simulink library "magField_custom_lib"  (R2018b)
settings: Solver=VariableStepAuto  StartTime=0.0  StopTime=10.0  RelTol=1e-3
settings Model: Creator=Taylor  LastModifiedBy=Taylor

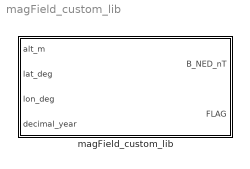
== system magField_custom_lib ==
  magField_custom_lib : Subsystem

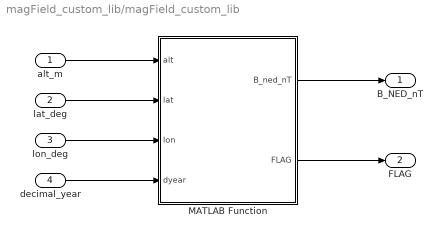
== system magField_custom_lib/magField_custom_lib ==
  alt_m : Inport
  lat_deg : Inport  Port=2
  lon_deg : Inport  Port=3
  decimal_year : Inport  Port=4
  MATLAB Function : MATLAB Function  TreatAsAtomicUnit=on
  B_NED_nT : Outport
  FLAG : Outport  Port=2
  wires:
  decimal_year/1 -> MATLAB Function/4(dyear)
  lon_deg/1 -> MATLAB Function/3(lon)
  lat_deg/1 -> MATLAB Function/2(lat)
  alt_m/1 -> MATLAB Function/1(alt)
  MATLAB Function/1(B_ned_nT) -> B_NED_nT/1
  MATLAB Function/2(FLAG) -> FLAG/1

== matlab function magField_custom_lib/MATLAB Function ==
  data: alt input; lat input; B_ned_nT output; lon input; dyear input; FLAG output
function [B_ned_nT,FLAG]  = my_wmm(alt,lat,lon,dyear)
%MY_WMM   World Magnetic Model
%
% B_NED_nT = my_wmm(lat,lon,alt,dyear) returns the magnetic field vector at
% the current latitude, longitude and altitude at the time specified by the 
% input dyear (decimal year). LLA can (should) be the output of the matlab
% function ecef2lla.m to make things simple. 
%
% Inputs:
%   - lat : geodetic latitude [degrees]
%   - lon : geodetic longitude [degrees]
%   - alt : altitude above the WGS84 ellipsoid [km]
%   - dyear : decimal year (e.g. 2016.25) MUST be greater than 2015.0
%
% Outputs: 
%   - B_ned_nT : magnetic field vector in the North-East-Down frame with
%   units of nanoTesla.
%   - FLAG : exit flag that indicates an error (-1) if the year is out of
%   range, otherwise this is 0.
%
% Current coefficients: WMM 2015v2 -- see Include/WMM_2015v2.COF file
% NOAA publishes user manuals, coefficient files and some software on their
% webiste here: https://www.ngdc.noaa.gov/geomag/WMM/soft.shtml#downloads
% This function was built from the WMM2015_Report.pdf 
%
% T. Reynolds -- RAIN Lab

%#codegen

% Constants
A       = 6378137;          % semi major axis [m]
a       = 6371200;          % geomagnetic reference radius
f       = 1/298.257223563;  % reciprocal flatening
e2      = f*(2-f);          % eccentricity squared
ord     = 12;               % model order 
maxord  = ord+1;
DEG2RAD = pi/180;

% HARD CODED COEFFICIENTS
t0 = 2015.0;
g = [ -29438.2, -1493.5,      0,      0,      0,     0,     0,     0,    0,     0,    0,    0, 0;
       -2444.5,  3014.7,   1679,      0,      0,     0,     0,     0,    0,     0,    0,    0, 0;
        1351.8, -2351.6, 1223.6,  582.3,      0,     0,     0,     0,    0,     0,    0,    0, 0;
         907.5,   814.8,  117.8, -335.6,   69.7,     0,     0,     0,    0,     0,    0,    0, 0;
        -232.9,   360.1,  191.7, -141.3, -157.2,   7.7,     0,     0,    0,     0,    0,    0, 0;
          69.4,    67.7,   72.3, -129.1,  -28.4,  13.6, -70.3,     0,    0,     0,    0,    0, 0;
          81.7,   -75.9,   -7.1,   52.2,   15,     9.1,    -3,   5.9,    0,     0,    0,    0, 0;
          24.2,     8.9,  -16.9,   -3.1,  -20.7,  13.3,  11.6, -16.3, -2.1,     0,    0,    0, 0;
           5.5,     8.8,      3,   -3.2,    0.6, -13.2,  -0.1,   8.7, -9.1, -10.4,    0,    0, 0;
            -2,    -6.1,    0.2,    0.6,   -0.5,   1.8,  -0.7,   2.2,  2.4,  -1.8, -3.6,    0, 0;
             3,    -1.4,   -2.3,    2.1,   -0.8,   0.6,  -0.7,   0.1,  1.7,  -0.2,  0.4,  3.5, 0;
            -2,    -0.1,    0.5,    1.2,   -0.9,   0.9,   0.1,   0.6, -0.4,  -0.5,  0.2, -0.9, 0 ];
     
h = [ 0,  4796.3,      0,      0,     0,     0,     0,    0,    0,    0,    0,    0, 0;
      0, -2842.4, -638.8,      0,     0,     0,     0,    0,    0,    0,    0,    0, 0;
      0,  -113.7,  246.5, -537.4,     0,     0,     0,    0,    0,    0,    0,    0, 0;
      0,   283.3, -188.6,  180.7,  -330,     0,     0,    0,    0,    0,    0,    0, 0;
      0,    46.9,  196.5, -119.9,    16, 100.6,     0,    0,    0,    0,    0,    0, 0;
      0,   -20.1,   32.8,   59.1, -67.1,   8.1,  61.9,    0,    0,    0,    0,    0, 0;
      0,   -54.3,  -19.5,      6,  24.5,   3.5, -27.7, -2.9,    0,    0,    0,    0, 0;
      0,    10.1,  -18.3,   13.3, -14.5,  16.2,     6, -9.2,  2.4,    0,    0,    0, 0;
      0,   -21.8,   10.7,   11.8,  -6.8,  -6.9,   7.9,    1, -3.9,  8.5,    0,    0, 0;
      0,     3.3,   -0.4,    4.6,   4.4,  -7.9,  -0.6, -4.2, -2.9, -1.1, -8.8,    0, 0;
      0,       0,    2.1,   -0.6,  -1.1,   0.7,  -0.2, -2.1, -1.5, -2.6,   -2, -2.3, 0;
      0,      -1,    0.3,    1.8,  -2.2,   0.3,   0.7, -0.1,  0.3,  0.2, -0.9, -0.2, 0.8 ];
  
dg = [    7,    9,    0,   0,    0,    0,    0,    0,    0,    0, 0,    0,  0;
        -11, -6.2,  0.3,   0,    0,    0,    0,    0,    0,    0, 0,    0,  0;
        2.4, -5.7,    2, -11,    0,    0,    0,    0,    0,    0, 0,    0,  0;
       -0.8, -0.9, -6.5, 5.2,   -4,    0,    0,    0,    0,    0, 0,    0,  0;
       -0.3,  0.6, -0.8, 0.1,  1.2,  1.4,    0,    0,    0,    0, 0,    0,  0;
       -0.8, -0.5, -0.1, 1.6, -1.6,    0,  1.2,    0,    0,    0, 0,    0,  0;
       -0.3, -0.2, -0.3, 0.9,  0.1, -0.6, -0.9,  0.7,    0,    0, 0,    0,  0;
       -0.1,  0.2, -0.2, 0.5, -0.1,  0.4,  0.4, -0.1,  0.4,    0, 0,    0,  0;
       -0.1, -0.1,    0, 0.4, -0.4,    0,  0.3,    0,    0, -0.3, 0,    0,  0;
        0,      0, -0.1, 0.2, -0.1, -0.2,    0, -0.1, -0.2, -0.1, 0,    0,  0;
        0,      0,    0,   0,    0, -0.1,    0,    0,    0, -0.1, 0, -0.1,  0;
        0,      0,    0,   0, -0.1,    0,    0,    0,    0,    0, 0,    0, -0.1 ];
    
dh = [ 0, -30.2,   0,    0,    0,    0,    0,    0,    0,    0,   0,   0,    0;
       0, -29.6, -17.3,  0,    0,    0,    0,    0,    0,    0,   0,   0,    0;
       0,   6.5,  -0.8, -2,    0,    0,    0,    0,    0,    0,   0,   0,    0;
       0,  -0.4,   5.8,  3.8, -3.5,  0,    0,    0,    0,    0,   0,   0,    0;
       0,   0.2,   2.3,  0,    3.3, -0.6,  0,    0,    0,    0,   0,   0,    0;
       0,   0.3,  -1.5, -1.2,  0.4,  0.2,  1.3,  0,    0,    0,   0,   0,    0;
       0,   0.6,   0.5, -0.8, -0.2, -1.1,  0.1,  0.2,  0,    0,   0,   0,    0;
       0,  -0.4,   0.6, -0.1,  0.6, -0.2, -0.5,  0.5,  0.1,  0,   0,   0,    0;
       0,  -0.3,   0.1, -0.4,  0.3,  0.1,  0,   -0.1,  0.5,  0.2, 0,   0,    0;
       0,   0,     0.1, -0.2,  0.1, -0.1,  0.1,  0,   -0.1,  0.2, 0,   0,    0;
       0,   0,     0.1,  0,    0.1,  0,    0,    0.1,  0,   -0.1, 0,  -0.1,  0;
       0,   0,     0,   -0.1,  0.1,  0,    0,    0,    0,    0,   0,   0,   -0.1 ];

% map inputs to right units
lat   = DEG2RAD * lat;
lon   = DEG2RAD * lon;
FLAG  = 0;
if (dyear < t0)
    FLAG = -1;
end
dt = dyear - t0;    % time since epoch
crlat = cos(lat);
srlat = sin(lat);
crlon = cos(lon);
srlon = sin(lon);

% clever recursive way of computing sin(m*lon) and cos(m*lon)
sp      = zeros(ord+1,1);
cp      = zeros(ord+1,1);
sp(2)   = srlon;
cp(1)   = 1.0; cp(2) = crlon;
for m=3:ord+1
    sp(m) = sp(2)*cp(m-1)+cp(2)*sp(m-1);
    cp(m) = cp(2)*cp(m-1)-sp(2)*sp(m-1);
end

% Step 1
Rc      = A/(sqrt(1-e2*srlat^2));   % normal section at latitude
p       = (Rc+alt) * crlat;
z       = (Rc*(1-e2)+alt)*srlat;
r       = sqrt(p^2+z^2);            % geocentric altitude
lat_gc  = asin(z/r);                % geocentric latitude
srlat   = sin(lat_gc);
aor     = a/r;                      % a over r
ar      = aor * aor;                % starts of squared, increases with n

% compute legendre polynomials
P   = zeros(maxord+1,maxord+1); % zeroth row and col added
x   = srlat;
xx  = sqrt(1-x*x);
trlat   = tan(lat_gc);
secrlat = sec(lat_gc);
P(1,1) = 1.0;           % this is P_0^0(x) = 1;
P(2,1) = x;             % this is P_1^0(x) = x;
P(2,2) = -xx;           % this is P_1^1(x) = -(1-x^2)^{1/2}
for n = 2:maxord    
    P(n+1,1) = (1/n)*(x*(2*n-1)*P(n,1) - (n-1)*P(n-1,1));
    for m = 1:n
        P(n+1,m+1) = (1/xx)*( (n-m+1)*x*P(n+1,m) - (n+m-1)*P(n,m) );
        if (m>1 && (n-m)>0)
            snorm = (-1)^(m-1) * sqrt(2*factorial(n-2-m+1)/factorial(n-2+m-1));
            P(n-1,m) = snorm * P(n-1,m);
        end
        if (m>1 && n==maxord)
            snorm = (-1)^(m-1) * sqrt(2*factorial(n-1-m+1)/factorial(n-1+m-1));
            P(n,m) = snorm * P(n,m);
            snorm = (-1)^(m-1) * sqrt(2*factorial(n-m+1)/factorial(n+m-1));
            P(n+1,m) = snorm * P(n+1,m);
        end
    end 
end
snorm = (-1)^(m) * sqrt(2*factorial(n-m)/factorial(n+m));
P(n+1,m+1) = snorm * P(n+1,m+1);

% Step 2 and 3 - main loop to compute components of B
bx = 0.0;
by = 0.0;
bz = 0.0;
for n = 1:ord
    ar    = ar * aor;
    for m = 0:n
        % derivative of lagrange polynomial P_n^m
        DPnm = (n+1)*trlat*P(n+1,m+1) - sqrt((n+1)^2-m^2)*secrlat*P(n+2,m+1);
        
        % adjust the Gauss coefficients for time elapsed since epoch
        G = g(n,m+1) + dt * dg(n,m+1);
        H = h(n,m+1) + dt * dh(n,m+1);
        
        % accumulate terms of spherical harmonic expansion
        bx = bx - ar * (G*cp(m+1)+H*sp(m+1))*DPnm;
        by = by + ar * m*(G*sp(m+1)-H*cp(m+1))*P(n+1,m+1);
        bz = bz - (n+1)*ar * (G*cp(m+1)+H*sp(m+1))*P(n+1,m+1);
        
    end
end

% Step 4 - rotate into the ellipsoidal reference frame
BX = bx*cos(lat_gc-lat) - bz*sin(lat_gc-lat);
BY = sec(lat_gc)*by;
BZ = bx*sin(lat_gc-lat) + bz*cos(lat_gc-lat);

% output final B vector
B_ned_nT = [BX; BY; BZ];

end
